simulink model "Filters"  (R2022a)
settings: Solver=FixedStepDiscrete  StartTime=0.0  StopTime=inf  RelTol=1e-3
InitFcn:
  | clear
  | addpath('./../1D/')
  | addpath(genpath('./nml'))
  | addpath('./MatLib')
  | 
  | % Run configuration file
  | [Beam, sBeam, modelSettings,...
  |         simulationSettings, plotSettings, simulinkSettings,...
  |         LO,KF,AKF,DKF,GDF,...
  |         Cd] = configure(1);
  | 
  | % Additional settings
  | AKF.nd = AKF.derivativeOrder;
  | DKF.nd = DKF.derivativeOrder;
  | modelSettings.l = 1;
  | 
  | % Build beam model, put it in model object
  | SYS = model();
  | [SYS, modelSettings] = buildBeam(modelSettings,simulationSettings,plotSettings,Beam,sBeam,SYS);
  | SYS.ny = size(SYS.dsys_sim,1);
  | SYS.nu = size(SYS.dsys_sim,2);
  | SYS.nq = size(SYS.dsys_sim.A,1);
  | 
  | SYS.dsys_obs = SYS.dsys_sim; %Because no error is introduced!
  | 
  | % Also initialise the filters in this model object
  | SYS = buildFilters(SYS,LO,KF,AKF,DKF,GDF);
  | 
  | % Some test matrices
  | Atest = eye(5);
  | Atest(1,5) = 15;
  | 
  | P0test = [ones(1,5);
  | ones(4,5)*2];
  | P0test(5,5) = 5;
undefined symbols (not defined in the file or in its folder): C28x, CPU1, CPU2
libraries: c2837xDlib x4, c2000lib x1
settings Model: SimulationMode=external  ExtModeTrigDuration=8  Creator=The MathWorks, Inc.  LastModifiedBy=pedeb
settings SolverCC: AlgebraicLoopSolver=TrustRegion  AutoInsertRateTranBlk=on
settings DataIOCC: LimitDataPoints=on  SaveFormat=Array  SaveOutput=off  SaveTime=off  ReturnWorkspaceOutputs=off
settings OptimizationCC: DefaultUnderspecifiedDataType=single  EnhancedBackFolding=on  MemcpyThreshold=512  PassReuseOutputArgsAs=Individual arguments  ExpressionDepthLimit=2147483647  ZeroExternalMemoryAtStartup=off  ZeroInternalMemoryAtStartup=off  MaxStackSize=64  OptimizeBlockOrder=speed  DifferentSizesBufferReuse=on  OptimizationCustomize=off  EfficientTunableParamExpr=on
settings DebuggingCC: UnderspecifiedInitializationDetection=Classic  MergeDetectMultiDrivingBlocksExec=none  SolverPrmCheckMsg=warning  MultiTaskDSMMsg=none  MultiTaskCondExecSysMsg=none  ParameterTunabilityLossMsg=error  FcnCallInpInsideContextMsg=warning  UnconnectedInputMsg=warning  UnconnectedOutputMsg=warning  UnconnectedLineMsg=warning  AllowSymbolicDim=off  StateNameClashWarn=warning  SFUnexpectedBacktrackingDiag=warning  SFNoUnconditionalDefaultTransitionDiag=warning  SFExecutionAtInitializationDiag=none  SFMachineParentedDataDiag=warning  ArithmeticOperatorsInVariantConditions=warning
settings HardwareCC: ProdBitPerChar=16  ProdBitPerInt=16  ProdBitPerPointer=32  ProdBitPerSizeT=32  ProdBitPerPtrDiffT=32  ProdLargestAtomicInteger=Integer  ProdLargestAtomicFloat=None  ProdWordSize=16  ProdHWDeviceType=Texas Instruments->C2000
settings ModelReferenceCC: PropagateSignalLabelsOutOfModel=off
settings SFSimCC: SimUseLocalCustomCode=off  MATLABDynamicMemAlloc=off  CustomCodeUndefinedFunction=UseInterfaceOnly  SimTargetLang=C++
settings RTWCC: SystemTargetFile=ert.tlc  HardwareBoard=TI Delfino F28379D LaunchPad  TemplateMakefile=ert_default_tmf  RTWVerbose=off  RTWUseLocalCustomCode=off  Toolchain=Texas Instruments Code Composer Studio (C2000)  BuildConfiguration=Specify  DLArmComputeVersion=19.05
settings CodeAppCC: ForceParamTrailComments=on  IgnoreCustomStorageClasses=off  OperatorAnnotations=on  SimulinkDataObjDesc=on  SFDataObjDesc=on  InsertBlockDesc=on
settings ERTTargetCC: InferredTypesCompatibility=on  SupportContinuousTime=on  SupportNonInlinedSFcns=on  ExtMode=on  ExtModeTransport=4  ExtModeStaticAlloc=on  ExtModeMexFile=ext_xcp  ExtModeMexArgs=1 14 5000000  ExtModeIntrfLevel=Level2 - Open
settings ConfigComp: CovMetricSettings=dw  CovSaveCumulativeToWorkspaceVar=on  CovSaveSingleToWorkspaceVar=on  CovExternalEMLEnable=off  CovSFcnEnable=off

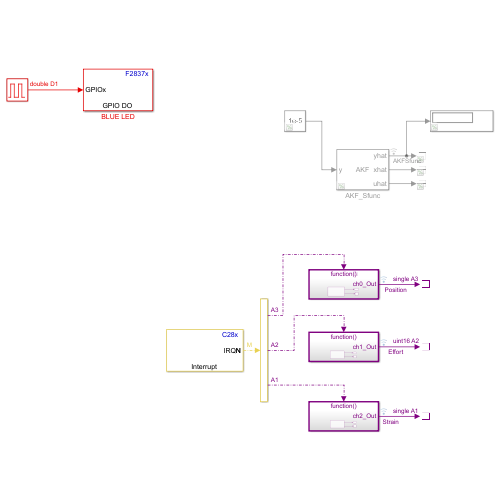
[thumbnail: Simulink's stored preview of the top-level diagram]
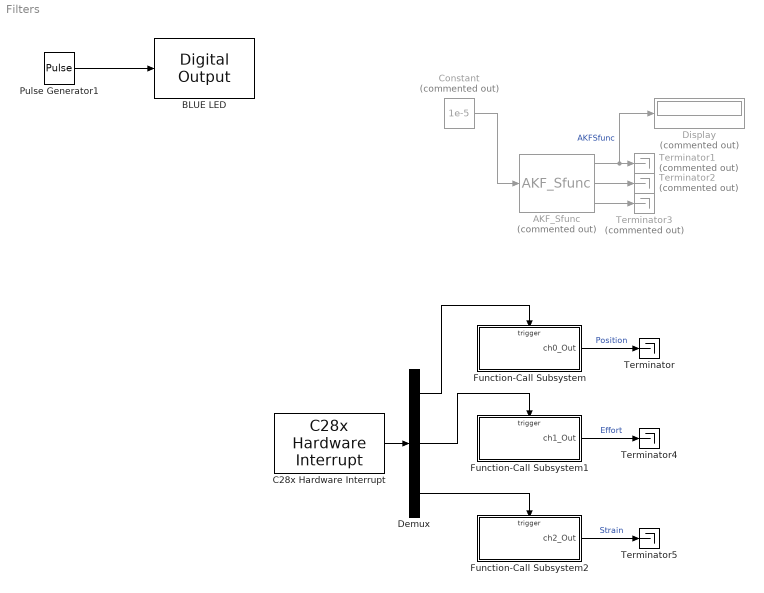
== system Filters ==
  AKF_Sfunc : S-Function  Commented=on  FunctionName=AKF_Sfunc  Parameters=Ap,Cp,Qp,Rp,Np,P0p,Bwp,nup,nyp,nqp  SFunctionDeploymentMode=off  EnableBusSupport=off  mask{Ap=SYS.AKF.A, Cp=SYS.AKF.C, Qp=SYS.AKF.Q, Rp=SYS.AKF.R, Np=SYS.AKF.S, P0p=SYS.AKF.P0_m, Bwp=SYS.AKF.Bw, nup=SYS.nu, nyp=SYS.ny, nqp=SYS.nq}
      mask prompts: Ap "A"; Cp "C"; Qp "Q"; Rp "R"; Np "N"; P0p "P0"; Bwp "Bw"; nup "nu"; nyp "ny"; nqp "nq"
      mask DialogControl DescGroupVar Prompt: AKF
      mask DialogControl DescTextVar Prompt: This block runs an Augmented Kalman filtering algorithm
      mask DialogControl Container4 Prompt: Model Sizes
      mask Display:
      | port_label('input', 1, 'y');
      | port_label('output', 1, 'yhat');
      | port_label('output', 2, 'xhat');
      | port_label('output', 3, 'uhat');
      | disp('AKF')
  BLUE LED : c2837xDlib/Digital Output  GPIO_Number=GPIO24~GPIO31  GPIO_Bit0=off  GPIO_BIT0_Toggle=off  GPIO_Bit1=off  GPIO_BIT1_Toggle=off  GPIO_Bit2=off  GPIO_BIT2_Toggle=off  GPIO_Bit3=off  GPIO_BIT3_Toggle=off  GPIO_Bit4=off  GPIO_BIT4_Toggle=off  GPIO_Bit5=off  GPIO_BIT5_Toggle=off  GPIO_Bit6=off  GPIO_BIT6_Toggle=off  GPIO_Bit7=on  GPIO_BIT7_Toggle=off
      settings: SourceProductBaseCode=TIC2000
  C28x Hardware Interrupt : c2000lib/Scheduling/C28x Hardware Interrupt  irqnumbers=[1 1 1]  pienumbers=[13 14 15]  irqpriorities=[30 29 28]  irqpreempts=[1 1 1]  showinput=off  dspchiptype=C280X
      settings: SourceProductBaseCode=TIC2000
  Constant : Constant  Commented=on  Value=1e-5  SampleTime=1/(1e3)
  Demux : Demux  Outputs=3
  Display : Display  Commented=on
  Function-Call Subsystem : Subsystem  TreatAsAtomicUnit=on
  Function-Call Subsystem1 : Subsystem  TreatAsAtomicUnit=on
  Function-Call Subsystem2 : Subsystem  TreatAsAtomicUnit=on
  Pulse Generator1 : DiscretePulseGenerator  PulseType=Time based  Period=1  PulseWidth=50  SampleTime=-1
  Terminator : Terminator
  Terminator1 : Terminator  Commented=on
  Terminator2 : Terminator  Commented=on
  Terminator3 : Terminator  Commented=on
  Terminator4 : Terminator
  Terminator5 : Terminator
  wires:
  Pulse Generator1/1 -> BLUE LED/1
  Constant/1 -> AKF_Sfunc/1
  AKF_Sfunc/1 -> Display/1, Terminator1/1  "AKFSfunc"
  AKF_Sfunc/2 -> Terminator2/1
  AKF_Sfunc/3 -> Terminator3/1
  Demux/2 -> Function-Call Subsystem1/Trigger
  Demux/1 -> Function-Call Subsystem/Trigger
  C28x Hardware Interrupt/1 -> Demux/1
  Function-Call Subsystem/1(ch0_Out) -> Terminator/1  "Position"
  Function-Call Subsystem1/1(ch1_Out) -> Terminator4/1  "Effort"
  Demux/3 -> Function-Call Subsystem2/Trigger
  Function-Call Subsystem2/1(ch2_Out) -> Terminator5/1  "Strain"

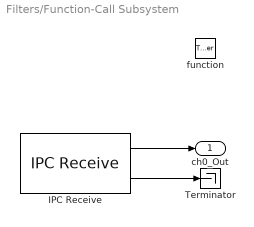
== system Filters/Function-Call Subsystem ==
  function : TriggerPort  TriggerType=function-call  VariantControl=Variant
  IPC Receive : c2837xDlib/IPC Receive  blkParamProc=F2837x  SelectSource=C28x (CPU1/CPU2)  SelectChannel=0  DataType=single  DataLength=1  EnableBlocking=off  SampleTime=-1
      settings: SourceProductBaseCode=TIC2000
  Terminator : Terminator
  ch0_Out : Outport
  wires:
  IPC Receive/2 -> Terminator/1
  IPC Receive/1 -> ch0_Out/1

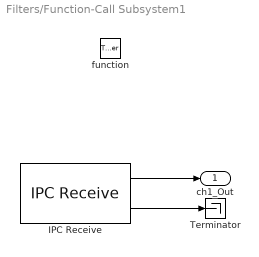
== system Filters/Function-Call Subsystem1 ==
  function : TriggerPort  TriggerType=function-call  VariantControl=Variant
  IPC Receive : c2837xDlib/IPC Receive  blkParamProc=F2837x  SelectSource=C28x (CPU1/CPU2)  SelectChannel=1  DataType=uint16  DataLength=1  EnableBlocking=off  SampleTime=-1
      settings: SourceProductBaseCode=TIC2000
  Terminator : Terminator
  ch1_Out : Outport
  wires:
  IPC Receive/2 -> Terminator/1
  IPC Receive/1 -> ch1_Out/1

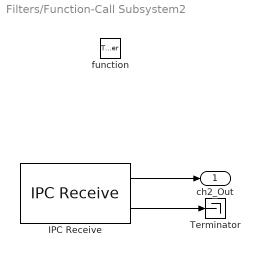
== system Filters/Function-Call Subsystem2 ==
  function : TriggerPort  TriggerType=function-call  VariantControl=Variant
  IPC Receive : c2837xDlib/IPC Receive  blkParamProc=F2837x  SelectSource=C28x (CPU1/CPU2)  SelectChannel=2  DataType=single  DataLength=1  EnableBlocking=off  SampleTime=-1
      settings: SourceProductBaseCode=TIC2000
  Terminator : Terminator
  ch2_Out : Outport
  wires:
  IPC Receive/1 -> ch2_Out/1
  IPC Receive/2 -> Terminator/1
